simulink model "x11"  (Simulink 7.2)
settings: Solver=ode45  StartTime=0.0  StopTime=10.0  RelTol=1e-3
libraries: cdsEpicsOut x289, cdsTP x288, cdsFilt x2, dac x2, cdsContec1616DIO x1, cdsParameters x1
(part 6 of 6)

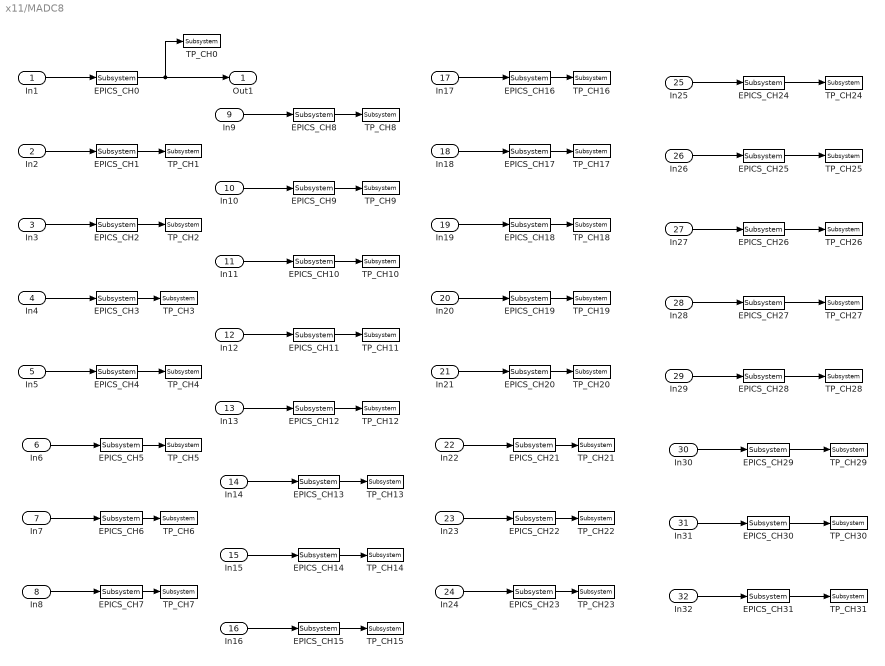
== system x11/MADC8 ==
  In1 : Inport  OutDataType=sfix(16)  OutScaling=2^0
  In2 : Inport  Port=2  OutDataType=sfix(16)  OutScaling=2^0
  In3 : Inport  Port=3  OutDataType=sfix(16)  OutScaling=2^0
  In4 : Inport  Port=4  OutDataType=sfix(16)  OutScaling=2^0
  In5 : Inport  Port=5  OutDataType=sfix(16)  OutScaling=2^0
  In6 : Inport  Port=6  OutDataType=sfix(16)  OutScaling=2^0
  In7 : Inport  Port=7  OutDataType=sfix(16)  OutScaling=2^0
  In8 : Inport  Port=8  OutDataType=sfix(16)  OutScaling=2^0
  In9 : Inport  Port=9  OutDataType=sfix(16)  OutScaling=2^0
  In10 : Inport  Port=10  OutDataType=sfix(16)  OutScaling=2^0
  In11 : Inport  Port=11  OutDataType=sfix(16)  OutScaling=2^0
  In12 : Inport  Port=12  OutDataType=sfix(16)  OutScaling=2^0
  In13 : Inport  Port=13  OutDataType=sfix(16)  OutScaling=2^0
  In14 : Inport  Port=14  OutDataType=sfix(16)  OutScaling=2^0
  In15 : Inport  Port=15  OutDataType=sfix(16)  OutScaling=2^0
  In16 : Inport  Port=16  OutDataType=sfix(16)  OutScaling=2^0
  In17 : Inport  Port=17  OutDataType=sfix(16)  OutScaling=2^0
  In18 : Inport  Port=18  OutDataType=sfix(16)  OutScaling=2^0
  In19 : Inport  Port=19  OutDataType=sfix(16)  OutScaling=2^0
  In20 : Inport  Port=20  OutDataType=sfix(16)  OutScaling=2^0
  In21 : Inport  Port=21  OutDataType=sfix(16)  OutScaling=2^0
  In22 : Inport  Port=22  OutDataType=sfix(16)  OutScaling=2^0
  In23 : Inport  Port=23  OutDataType=sfix(16)  OutScaling=2^0
  In24 : Inport  Port=24  OutDataType=sfix(16)  OutScaling=2^0
  In25 : Inport  Port=25  OutDataType=sfix(16)  OutScaling=2^0
  In26 : Inport  Port=26  OutDataType=sfix(16)  OutScaling=2^0
  In27 : Inport  Port=27  OutDataType=sfix(16)  OutScaling=2^0
  In28 : Inport  Port=28  OutDataType=sfix(16)  OutScaling=2^0
  In29 : Inport  Port=29  OutDataType=sfix(16)  OutScaling=2^0
  In30 : Inport  Port=30  OutDataType=sfix(16)  OutScaling=2^0
  In31 : Inport  Port=31  OutDataType=sfix(16)  OutScaling=2^0
  In32 : Inport  Port=32  OutDataType=sfix(16)  OutScaling=2^0
  EPICS_CH0 : cdsEpicsOut/Subsystem  Tag=cdsEpicsOutput  Description=|  SystemSampleTime=-1
      | Purpose:                                          
      | Output a FE signal to an EPICS channel.           
      |                                                   
      | Operation:                                        
      | Takes input value and passes it to EPICS record.  
      |                                                   
      | Usage:                                            
      | Name the part with the desired EPICS rrecord name.
      settings: AttributesFormatString=%<Tag>
  EPICS_CH1 : cdsEpicsOut/Subsystem  Tag=cdsEpicsOutput  Description=|  SystemSampleTime=-1
      | Purpose:                                          
      | Output a FE signal to an EPICS channel.           
      |                                                   
      | Operation:                                        
      | Takes input value and passes it to EPICS record.  
      |                                                   
      | Usage:                                            
      | Name the part with the desired EPICS rrecord name.
      settings: AttributesFormatString=%<Tag>
  EPICS_CH10 : cdsEpicsOut/Subsystem  Tag=cdsEpicsOutput  Description=|  SystemSampleTime=-1
      | Purpose:                                          
      | Output a FE signal to an EPICS channel.           
      |                                                   
      | Operation:                                        
      | Takes input value and passes it to EPICS record.  
      |                                                   
      | Usage:                                            
      | Name the part with the desired EPICS rrecord name.
      settings: AttributesFormatString=%<Tag>
  EPICS_CH11 : cdsEpicsOut/Subsystem  Tag=cdsEpicsOutput  Description=|  SystemSampleTime=-1
      | Purpose:                                          
      | Output a FE signal to an EPICS channel.           
      |                                                   
      | Operation:                                        
      | Takes input value and passes it to EPICS record.  
      |                                                   
      | Usage:                                            
      | Name the part with the desired EPICS rrecord name.
      settings: AttributesFormatString=%<Tag>
  EPICS_CH12 : cdsEpicsOut/Subsystem  Tag=cdsEpicsOutput  Description=|  SystemSampleTime=-1
      | Purpose:                                          
      | Output a FE signal to an EPICS channel.           
      |                                                   
      | Operation:                                        
      | Takes input value and passes it to EPICS record.  
      |                                                   
      | Usage:                                            
      | Name the part with the desired EPICS rrecord name.
      settings: AttributesFormatString=%<Tag>
  EPICS_CH13 : cdsEpicsOut/Subsystem  Tag=cdsEpicsOutput  Description=|  SystemSampleTime=-1
      | Purpose:                                          
      | Output a FE signal to an EPICS channel.           
      |                                                   
      | Operation:                                        
      | Takes input value and passes it to EPICS record.  
      |                                                   
      | Usage:                                            
      | Name the part with the desired EPICS rrecord name.
      settings: AttributesFormatString=%<Tag>
  EPICS_CH14 : cdsEpicsOut/Subsystem  Tag=cdsEpicsOutput  Description=|  SystemSampleTime=-1
      | Purpose:                                          
      | Output a FE signal to an EPICS channel.           
      |                                                   
      | Operation:                                        
      | Takes input value and passes it to EPICS record.  
      |                                                   
      | Usage:                                            
      | Name the part with the desired EPICS rrecord name.
      settings: AttributesFormatString=%<Tag>
  EPICS_CH15 : cdsEpicsOut/Subsystem  Tag=cdsEpicsOutput  Description=|  SystemSampleTime=-1
      | Purpose:                                          
      | Output a FE signal to an EPICS channel.           
      |                                                   
      | Operation:                                        
      | Takes input value and passes it to EPICS record.  
      |                                                   
      | Usage:                                            
      | Name the part with the desired EPICS rrecord name.
      settings: AttributesFormatString=%<Tag>
  EPICS_CH16 : cdsEpicsOut/Subsystem  Tag=cdsEpicsOutput  Description=|  SystemSampleTime=-1
      | Purpose:                                          
      | Output a FE signal to an EPICS channel.           
      |                                                   
      | Operation:                                        
      | Takes input value and passes it to EPICS record.  
      |                                                   
      | Usage:                                            
      | Name the part with the desired EPICS rrecord name.
      settings: AttributesFormatString=%<Tag>
  EPICS_CH17 : cdsEpicsOut/Subsystem  Tag=cdsEpicsOutput  Description=|  SystemSampleTime=-1
      | Purpose:                                          
      | Output a FE signal to an EPICS channel.           
      |                                                   
      | Operation:                                        
      | Takes input value and passes it to EPICS record.  
      |                                                   
      | Usage:                                            
      | Name the part with the desired EPICS rrecord name.
      settings: AttributesFormatString=%<Tag>
  EPICS_CH18 : cdsEpicsOut/Subsystem  Tag=cdsEpicsOutput  Description=|  SystemSampleTime=-1
      | Purpose:                                          
      | Output a FE signal to an EPICS channel.           
      |                                                   
      | Operation:                                        
      | Takes input value and passes it to EPICS record.  
      |                                                   
      | Usage:                                            
      | Name the part with the desired EPICS rrecord name.
      settings: AttributesFormatString=%<Tag>
  EPICS_CH19 : cdsEpicsOut/Subsystem  Tag=cdsEpicsOutput  Description=|  SystemSampleTime=-1
      | Purpose:                                          
      | Output a FE signal to an EPICS channel.           
      |                                                   
      | Operation:                                        
      | Takes input value and passes it to EPICS record.  
      |                                                   
      | Usage:                                            
      | Name the part with the desired EPICS rrecord name.
      settings: AttributesFormatString=%<Tag>
  EPICS_CH2 : cdsEpicsOut/Subsystem  Tag=cdsEpicsOutput  Description=|  SystemSampleTime=-1
      | Purpose:                                          
      | Output a FE signal to an EPICS channel.           
      |                                                   
      | Operation:                                        
      | Takes input value and passes it to EPICS record.  
      |                                                   
      | Usage:                                            
      | Name the part with the desired EPICS rrecord name.
      settings: AttributesFormatString=%<Tag>
  EPICS_CH20 : cdsEpicsOut/Subsystem  Tag=cdsEpicsOutput  Description=|  SystemSampleTime=-1
      | Purpose:                                          
      | Output a FE signal to an EPICS channel.           
      |                                                   
      | Operation:                                        
      | Takes input value and passes it to EPICS record.  
      |                                                   
      | Usage:                                            
      | Name the part with the desired EPICS rrecord name.
      settings: AttributesFormatString=%<Tag>
  EPICS_CH21 : cdsEpicsOut/Subsystem  Tag=cdsEpicsOutput  Description=|  SystemSampleTime=-1
      | Purpose:                                          
      | Output a FE signal to an EPICS channel.           
      |                                                   
      | Operation:                                        
      | Takes input value and passes it to EPICS record.  
      |                                                   
      | Usage:                                            
      | Name the part with the desired EPICS rrecord name.
      settings: AttributesFormatString=%<Tag>
  EPICS_CH22 : cdsEpicsOut/Subsystem  Tag=cdsEpicsOutput  Description=|  SystemSampleTime=-1
      | Purpose:                                          
      | Output a FE signal to an EPICS channel.           
      |                                                   
      | Operation:                                        
      | Takes input value and passes it to EPICS record.  
      |                                                   
      | Usage:                                            
      | Name the part with the desired EPICS rrecord name.
      settings: AttributesFormatString=%<Tag>
  EPICS_CH23 : cdsEpicsOut/Subsystem  Tag=cdsEpicsOutput  Description=|  SystemSampleTime=-1
      | Purpose:                                          
      | Output a FE signal to an EPICS channel.           
      |                                                   
      | Operation:                                        
      | Takes input value and passes it to EPICS record.  
      |                                                   
      | Usage:                                            
      | Name the part with the desired EPICS rrecord name.
      settings: AttributesFormatString=%<Tag>
  EPICS_CH24 : cdsEpicsOut/Subsystem  Tag=cdsEpicsOutput  Description=|  SystemSampleTime=-1
      | Purpose:                                          
      | Output a FE signal to an EPICS channel.           
      |                                                   
      | Operation:                                        
      | Takes input value and passes it to EPICS record.  
      |                                                   
      | Usage:                                            
      | Name the part with the desired EPICS rrecord name.
      settings: AttributesFormatString=%<Tag>
  EPICS_CH25 : cdsEpicsOut/Subsystem  Tag=cdsEpicsOutput  Description=|  SystemSampleTime=-1
      | Purpose:                                          
      | Output a FE signal to an EPICS channel.           
      |                                                   
      | Operation:                                        
      | Takes input value and passes it to EPICS record.  
      |                                                   
      | Usage:                                            
      | Name the part with the desired EPICS rrecord name.
      settings: AttributesFormatString=%<Tag>
  EPICS_CH26 : cdsEpicsOut/Subsystem  Tag=cdsEpicsOutput  Description=|  SystemSampleTime=-1
      | Purpose:                                          
      | Output a FE signal to an EPICS channel.           
      |                                                   
      | Operation:                                        
      | Takes input value and passes it to EPICS record.  
      |                                                   
      | Usage:                                            
      | Name the part with the desired EPICS rrecord name.
      settings: AttributesFormatString=%<Tag>
  EPICS_CH27 : cdsEpicsOut/Subsystem  Tag=cdsEpicsOutput  Description=|  SystemSampleTime=-1
      | Purpose:                                          
      | Output a FE signal to an EPICS channel.           
      |                                                   
      | Operation:                                        
      | Takes input value and passes it to EPICS record.  
      |                                                   
      | Usage:                                            
      | Name the part with the desired EPICS rrecord name.
      settings: AttributesFormatString=%<Tag>
  EPICS_CH28 : cdsEpicsOut/Subsystem  Tag=cdsEpicsOutput  Description=|  SystemSampleTime=-1
      | Purpose:                                          
      | Output a FE signal to an EPICS channel.           
      |                                                   
      | Operation:                                        
      | Takes input value and passes it to EPICS record.  
      |                                                   
      | Usage:                                            
      | Name the part with the desired EPICS rrecord name.
      settings: AttributesFormatString=%<Tag>
  EPICS_CH29 : cdsEpicsOut/Subsystem  Tag=cdsEpicsOutput  Description=|  SystemSampleTime=-1
      | Purpose:                                          
      | Output a FE signal to an EPICS channel.           
      |                                                   
      | Operation:                                        
      | Takes input value and passes it to EPICS record.  
      |                                                   
      | Usage:                                            
      | Name the part with the desired EPICS rrecord name.
      settings: AttributesFormatString=%<Tag>
  EPICS_CH3 : cdsEpicsOut/Subsystem  Tag=cdsEpicsOutput  Description=|  SystemSampleTime=-1
      | Purpose:                                          
      | Output a FE signal to an EPICS channel.           
      |                                                   
      | Operation:                                        
      | Takes input value and passes it to EPICS record.  
      |                                                   
      | Usage:                                            
      | Name the part with the desired EPICS rrecord name.
      settings: AttributesFormatString=%<Tag>
  EPICS_CH30 : cdsEpicsOut/Subsystem  Tag=cdsEpicsOutput  Description=|  SystemSampleTime=-1
      | Purpose:                                          
      | Output a FE signal to an EPICS channel.           
      |                                                   
      | Operation:                                        
      | Takes input value and passes it to EPICS record.  
      |                                                   
      | Usage:                                            
      | Name the part with the desired EPICS rrecord name.
      settings: AttributesFormatString=%<Tag>
  EPICS_CH31 : cdsEpicsOut/Subsystem  Tag=cdsEpicsOutput  Description=|  SystemSampleTime=-1
      | Purpose:                                          
      | Output a FE signal to an EPICS channel.           
      |                                                   
      | Operation:                                        
      | Takes input value and passes it to EPICS record.  
      |                                                   
      | Usage:                                            
      | Name the part with the desired EPICS rrecord name.
      settings: AttributesFormatString=%<Tag>
  EPICS_CH4 : cdsEpicsOut/Subsystem  Tag=cdsEpicsOutput  Description=|  SystemSampleTime=-1
      | Purpose:                                          
      | Output a FE signal to an EPICS channel.           
      |                                                   
      | Operation:                                        
      | Takes input value and passes it to EPICS record.  
      |                                                   
      | Usage:                                            
      | Name the part with the desired EPICS rrecord name.
      settings: AttributesFormatString=%<Tag>
  EPICS_CH5 : cdsEpicsOut/Subsystem  Tag=cdsEpicsOutput  Description=|  SystemSampleTime=-1
      | Purpose:                                          
      | Output a FE signal to an EPICS channel.           
      |                                                   
      | Operation:                                        
      | Takes input value and passes it to EPICS record.  
      |                                                   
      | Usage:                                            
      | Name the part with the desired EPICS rrecord name.
      settings: AttributesFormatString=%<Tag>
  EPICS_CH6 : cdsEpicsOut/Subsystem  Tag=cdsEpicsOutput  Description=|  SystemSampleTime=-1
      | Purpose:                                          
      | Output a FE signal to an EPICS channel.           
      |                                                   
      | Operation:                                        
      | Takes input value and passes it to EPICS record.  
      |                                                   
      | Usage:                                            
      | Name the part with the desired EPICS rrecord name.
      settings: AttributesFormatString=%<Tag>
  EPICS_CH7 : cdsEpicsOut/Subsystem  Tag=cdsEpicsOutput  Description=|  SystemSampleTime=-1
      | Purpose:                                          
      | Output a FE signal to an EPICS channel.           
      |                                                   
      | Operation:                                        
      | Takes input value and passes it to EPICS record.  
      |                                                   
      | Usage:                                            
      | Name the part with the desired EPICS rrecord name.
      settings: AttributesFormatString=%<Tag>
  EPICS_CH8 : cdsEpicsOut/Subsystem  Tag=cdsEpicsOutput  Description=|  SystemSampleTime=-1
      | Purpose:                                          
      | Output a FE signal to an EPICS channel.           
      |                                                   
      | Operation:                                        
      | Takes input value and passes it to EPICS record.  
      |                                                   
      | Usage:                                            
      | Name the part with the desired EPICS rrecord name.
      settings: AttributesFormatString=%<Tag>
  EPICS_CH9 : cdsEpicsOut/Subsystem  Tag=cdsEpicsOutput  Description=|  SystemSampleTime=-1
      | Purpose:                                          
      | Output a FE signal to an EPICS channel.           
      |                                                   
      | Operation:                                        
      | Takes input value and passes it to EPICS record.  
      |                                                   
      | Usage:                                            
      | Name the part with the desired EPICS rrecord name.
      settings: AttributesFormatString=%<Tag>
  TP_CH{0..31} (32 alike) : cdsTP/Subsystem  Tag=Test Point  SystemSampleTime=-1
      settings: AttributesFormatString=%<Tag>
  Out1 : Outport  OutDataType=sfix(16)  OutScaling=2^0
  wires:
  In1/1 -> EPICS_CH0/1
  EPICS_CH0/1 -> Out1/1, TP_CH0/1
  In2/1 -> EPICS_CH1/1
  In3/1 -> EPICS_CH2/1
  In4/1 -> EPICS_CH3/1
  In5/1 -> EPICS_CH4/1
  In6/1 -> EPICS_CH5/1
  In7/1 -> EPICS_CH6/1
  In8/1 -> EPICS_CH7/1
  In9/1 -> EPICS_CH8/1
  In10/1 -> EPICS_CH9/1
  In11/1 -> EPICS_CH10/1
  In12/1 -> EPICS_CH11/1
  In13/1 -> EPICS_CH12/1
  In14/1 -> EPICS_CH13/1
  In15/1 -> EPICS_CH14/1
  In16/1 -> EPICS_CH15/1
  In17/1 -> EPICS_CH16/1
  In18/1 -> EPICS_CH17/1
  In19/1 -> EPICS_CH18/1
  In20/1 -> EPICS_CH19/1
  In21/1 -> EPICS_CH20/1
  In22/1 -> EPICS_CH21/1
  In23/1 -> EPICS_CH22/1
  In24/1 -> EPICS_CH23/1
  In25/1 -> EPICS_CH24/1
  In26/1 -> EPICS_CH25/1
  In27/1 -> EPICS_CH26/1
  In28/1 -> EPICS_CH27/1
  In29/1 -> EPICS_CH28/1
  In30/1 -> EPICS_CH29/1
  In31/1 -> EPICS_CH30/1
  In32/1 -> EPICS_CH31/1
  EPICS_CH1/1 -> TP_CH1/1
  EPICS_CH2/1 -> TP_CH2/1
  EPICS_CH3/1 -> TP_CH3/1
  EPICS_CH4/1 -> TP_CH4/1
  EPICS_CH5/1 -> TP_CH5/1
  EPICS_CH6/1 -> TP_CH6/1
  EPICS_CH7/1 -> TP_CH7/1
  EPICS_CH8/1 -> TP_CH8/1
  EPICS_CH9/1 -> TP_CH9/1
  EPICS_CH10/1 -> TP_CH10/1
  EPICS_CH11/1 -> TP_CH11/1
  EPICS_CH12/1 -> TP_CH12/1
  EPICS_CH13/1 -> TP_CH13/1
  EPICS_CH14/1 -> TP_CH14/1
  EPICS_CH15/1 -> TP_CH15/1
  EPICS_CH16/1 -> TP_CH16/1
  EPICS_CH17/1 -> TP_CH17/1
  EPICS_CH18/1 -> TP_CH18/1
  EPICS_CH19/1 -> TP_CH19/1
  EPICS_CH20/1 -> TP_CH20/1
  EPICS_CH21/1 -> TP_CH21/1
  EPICS_CH22/1 -> TP_CH22/1
  EPICS_CH23/1 -> TP_CH23/1
  EPICS_CH24/1 -> TP_CH24/1
  EPICS_CH25/1 -> TP_CH25/1
  EPICS_CH26/1 -> TP_CH26/1
  EPICS_CH27/1 -> TP_CH27/1
  EPICS_CH28/1 -> TP_CH28/1
  EPICS_CH29/1 -> TP_CH29/1
  EPICS_CH30/1 -> TP_CH30/1
  EPICS_CH31/1 -> TP_CH31/1
